simulink model "sepic_sic_pv"  (R2025b)
settings: Solver=FixedStepDiscrete  StartTime=0.0  StopTime=0.025  FixedStep=5e-08  RelTol=1e-3
libraries: spsSeriesRLCBranchLib x9, spsDiodeLib x4, spsVoltageMeasurementLib x4, spsCurrentMeasurementLib x2, spsPVArrayLib x1, spsMosfetLib x1, spspowerguiLib x1
settings Model: Creator=artes  LastModifiedBy=artes

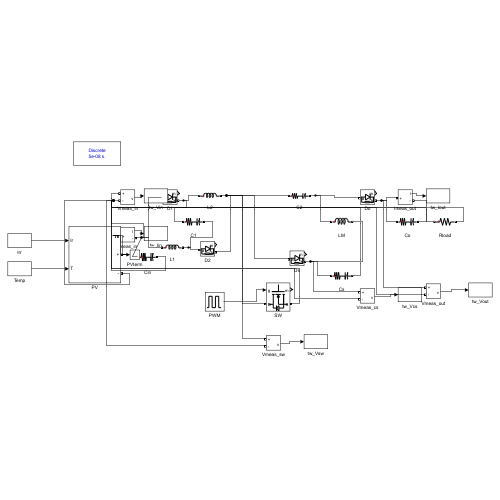
[thumbnail: Simulink's stored preview of the top-level diagram]
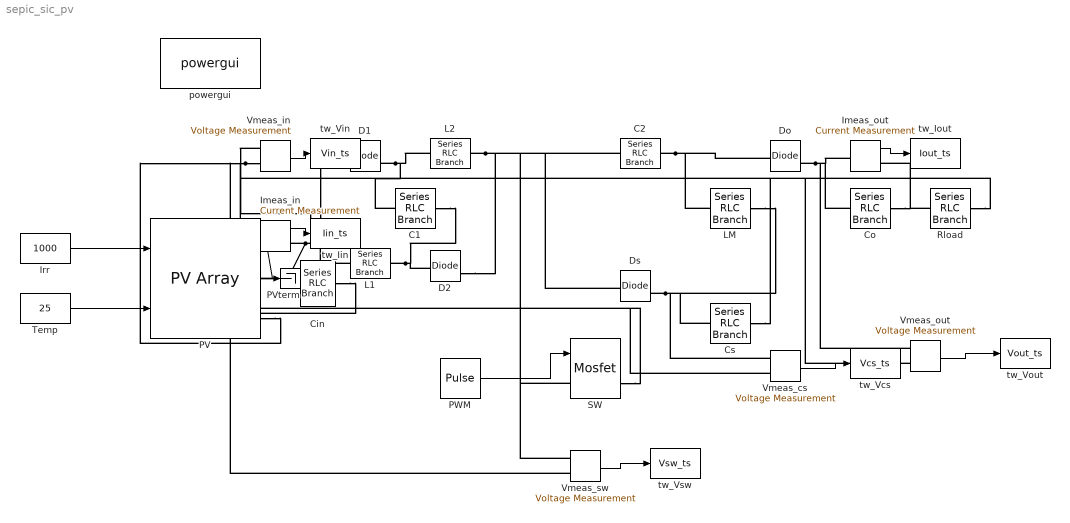
== system sepic_sic_pv ==
  C1 : spsSeriesRLCBranchLib/Series RLC Branch  LConnTagsString=__new0  RConnTagsString=__new0  BranchType=RC  Resistance=0.03  Inductance=1e-3  SetiL0=off  InitialCurrent=0  Capacitance=4.7e-05  Setx0=off  InitialVoltage=0  Measurements=None
  C2 : spsSeriesRLCBranchLib/Series RLC Branch  LConnTagsString=__new0  RConnTagsString=__new0  BranchType=RC  Resistance=0.03  Inductance=1e-3  SetiL0=off  InitialCurrent=0  Capacitance=2.2e-05  Setx0=off  InitialVoltage=0  Measurements=None
  Cin : spsSeriesRLCBranchLib/Series RLC Branch  LConnTagsString=__new0  RConnTagsString=__new0  BranchType=RC  Resistance=0.02  Inductance=1e-3  SetiL0=off  InitialCurrent=0  Capacitance=100e-6  Setx0=off  InitialVoltage=0  Measurements=None
  Co : spsSeriesRLCBranchLib/Series RLC Branch  LConnTagsString=__new0  RConnTagsString=__new0  BranchType=RC  Resistance=0.03  Inductance=1e-3  SetiL0=off  InitialCurrent=0  Capacitance=2.2e-05  Setx0=off  InitialVoltage=0  Measurements=None
  Cs : spsSeriesRLCBranchLib/Series RLC Branch  LConnTagsString=__new0  RConnTagsString=__new0  BranchType=RC  Resistance=0.03  Inductance=1e-3  SetiL0=off  InitialCurrent=0  Capacitance=1e-05  Setx0=off  InitialVoltage=0  Measurements=None
  D1 : spsDiodeLib/Diode  Ron=0.001  Lon=0  Vf=0.8  IC=0  UseSnubber=0  Rs=500  Cs=250e-9  Measurements=on
  D2 : spsDiodeLib/Diode  Ron=0.001  Lon=0  Vf=0.8  IC=0  UseSnubber=0  Rs=500  Cs=250e-9  Measurements=on
  Do : spsDiodeLib/Diode  Ron=0.001  Lon=0  Vf=0.8  IC=0  UseSnubber=0  Rs=500  Cs=250e-9  Measurements=on
  Ds : spsDiodeLib/Diode  Ron=0.001  Lon=0  Vf=0.8  IC=0  UseSnubber=0  Rs=500  Cs=250e-9  Measurements=on
  Imeas_in : spsCurrentMeasurementLib/Current Measurement  PhasorSimulation=off  OutputType=Complex  PSBequivalent=0
  Imeas_out : spsCurrentMeasurementLib/Current Measurement  PhasorSimulation=off  OutputType=Complex  PSBequivalent=0
  Irr : Constant  Value=1000
  L1 : spsSeriesRLCBranchLib/Series RLC Branch  LConnTagsString=__new0  RConnTagsString=__new0  BranchType=L  Resistance=1  Inductance=0.00015  SetiL0=off  InitialCurrent=0  Capacitance=1e-6  Setx0=off  InitialVoltage=0  Measurements=None
  L2 : spsSeriesRLCBranchLib/Series RLC Branch  LConnTagsString=__new0  RConnTagsString=__new0  BranchType=L  Resistance=1  Inductance=0.00015  SetiL0=off  InitialCurrent=0  Capacitance=1e-6  Setx0=off  InitialVoltage=0  Measurements=None
  LM : spsSeriesRLCBranchLib/Series RLC Branch  LConnTagsString=__new0  RConnTagsString=__new0  BranchType=L  Resistance=1  Inductance=0.00033  SetiL0=off  InitialCurrent=0  Capacitance=1e-6  Setx0=off  InitialVoltage=0  Measurements=None
  PV : spsPVArrayLib/PV Array  Npar=1  Nser=1  PlotType=array @ 1000 W/m2 & specified temperatures  S_vec="[ 1000  500  100 ]"  Temp_C_vec="[ 45 25  ]"  ModuleName=User-defined  PlotWhenSelected=off  Pm=448.8  Ncell=72  Voc=40  Isc=13.9  Vm=34  Im=13.2  beta_Voc_pc=-0.36099  alpha_Isc_pc=0.102  beta_Voc=-0.1444  alpha_Isc=0.014178  IL=13.9443  I0=5.1999e-10  nI=0.90078  Rsh=408.9693  Rs=0.070544  RobustModel=off  RobustCellTemperature=313.3991  BAL=on  Tc=1e-6  Tfilter=5e-5
  PVterm : Terminator
  PWM : DiscretePulseGenerator  PulseType=Time based  Period=2e-05  PulseWidth=51.25
  Rload : spsSeriesRLCBranchLib/Series RLC Branch  LConnTagsString=__new0  RConnTagsString=__new0  BranchType=R  Resistance=100  Inductance=1e-3  SetiL0=off  InitialCurrent=0  Capacitance=1e-6  Setx0=off  InitialVoltage=0  Measurements=None
  SW : spsMosfetLib/Mosfet  Ron=0.02  Lon=0  Rd=0.01  Vfd=0  IC=0  Rs=1e5  Cs=inf  Measurements=on
  Temp : Constant  Value=25
  Vmeas_cs : spsVoltageMeasurementLib/Voltage Measurement  PhasorSimulation=off  OutputType=Complex  PSBequivalent=0
  Vmeas_in : spsVoltageMeasurementLib/Voltage Measurement  PhasorSimulation=off  OutputType=Complex  PSBequivalent=0
  Vmeas_out : spsVoltageMeasurementLib/Voltage Measurement  PhasorSimulation=off  OutputType=Complex  PSBequivalent=0
  Vmeas_sw : spsVoltageMeasurementLib/Voltage Measurement  PhasorSimulation=off  OutputType=Complex  PSBequivalent=0
  powergui : spspowerguiLib/powergui  Priority=1  SimulationMode=Discrete  SampleTime=5e-08  frequency=60  Iterations=50  frequencyindice=60  Pbase=100e6  ErrMax=1e-4  UnitsV=kV  UnitsW=MW  buscounter=0  FunctionMessages=off  echomessages=off  EnableUseOfTLC=off  CurrentSourceSwitches=off  DisableSnubberDevices=off  DisableRonSwitches=off  DisableVfSwitches=off  DisplayEquations=off  AutomaticDiscreteSolvers=off  SolverType=Tustin/Backward Euler (TBE)  Interpol=off  ExternalGateDelay=off  methode=off  Ts=100  x0status=blocks  SPID=on  SwTol=0  HookPort=off  NonlinearTolerance=1e-4  nMaxIteration=100  ContinueOnMaxIteration=off  RestoreLinks=warning  ResistiveCurrentMeasurement=off  Frange=[0:2:500]  Ylog=off  Xlog=on  ShowGrid=off  save=off  variable=ZData  structure=0  ZoomFFT=off  StartTime=0.0  cycles=1  DisplayStyle=1  fundamental=60  FreqAxis=off  MaxFrequency=1000  frequencyindicesteady=1  RmsSteady=1  display=off
  tw_Iin : ToWorkspace  VariableName=Iin_ts  SaveFormat=Timeseries  SampleTime=-1
  tw_Iout : ToWorkspace  VariableName=Iout_ts  SaveFormat=Timeseries  SampleTime=-1
  tw_Vcs : ToWorkspace  VariableName=Vcs_ts  SaveFormat=Timeseries  SampleTime=-1
  tw_Vin : ToWorkspace  VariableName=Vin_ts  SaveFormat=Timeseries  SampleTime=-1
  tw_Vout : ToWorkspace  VariableName=Vout_ts  SaveFormat=Timeseries  SampleTime=-1
  tw_Vsw : ToWorkspace  VariableName=Vsw_ts  SaveFormat=Timeseries  SampleTime=-1
  wires:
  PWM/1 -> SW/1
  Vmeas_out/1 -> tw_Vout/1
  Imeas_out/1 -> tw_Iout/1
  Imeas_in/1 -> tw_Iin/1
  Vmeas_in/1 -> tw_Vin/1
  Vmeas_cs/1 -> tw_Vcs/1
  Vmeas_sw/1 -> tw_Vsw/1
  Irr/1 -> PV/1
  Temp/1 -> PV/2
  PV/1 -> PVterm/1
  connections:
  Vmeas_in/LConn1 -- D1/LConn1 -- L1/LConn1 -- Imeas_in/RConn1 -- Cin/LConn1
  D1/RConn1 -- L2/LConn1 -- C1/LConn1
  L1/RConn1 -- D2/LConn1 -- C1/RConn1
  D2/RConn1 -- SW/LConn1 -- Ds/LConn1 -- C2/LConn1 -- L2/RConn1 -- Vmeas_sw/LConn1
  SW/RConn1 -- Cs/RConn1 -- Co/RConn1 -- Rload/RConn1 -- Vmeas_out/LConn2 -- Vmeas_cs/LConn2 -- Vmeas_sw/LConn2 -- Cin/RConn1 -- Vmeas_in/LConn2 -- PV/RConn2
  C2/RConn1 -- LM/LConn1 -- Do/LConn1
  LM/RConn1 -- Cs/LConn1 -- Ds/RConn1 -- Vmeas_cs/LConn1
  Co/LConn1 -- Imeas_out/LConn1 -- Do/RConn1 -- Vmeas_out/LConn1
  Rload/LConn1 -- Imeas_out/RConn1
  PV/RConn1 -- Imeas_in/LConn1
